simulink model "gm_uz_pmsm_model_9ph_vnl"  (R2021b)
settings: Solver=FixedStepAuto  StartTime=0.0  StopTime=0.8  RelTol=1e-3
PreLoadFcn:
  | uz_pmsm_model_9ph_init_parameter
undefined symbols (not defined in the file or in its folder): a, b, c, friction_coefficient, inertia, k_i_d, k_i_q, k_p_d, k_p_q, Kpd, L_d, L_o1, L_o2, L_q, L_x1, L_x2, L_y1, L_y2, L_zero, polepair, psi_pm, R_1, static_friction_torque, Tnd, ts
libraries: hdlmdlgenlib x191, hdlsllib x90, dspsigops x19, simulink x17, slpidlib x2, spsAlphaBetaZerotodq0Lib x1, pid_lib x1, spsdq0toAlphaBetaZeroLib x1
(part 2 of 7)

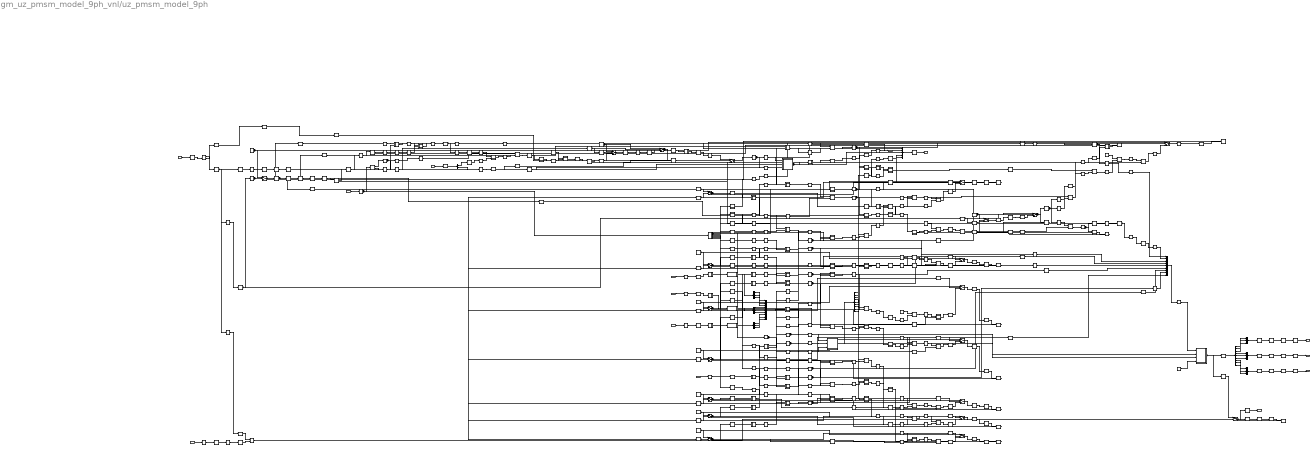
== system gm_uz_pmsm_model_9ph_vnl/uz_pmsm_model_9ph ==
  note: PMSM electric and magentic
  note: Mechanical
  note: Outputs
  note: Inputs
  note: o1 equation
  note: DQ equations
  note: o2 equation
  note: x1 equation
  note: y1 equation
  note: x2 equation
  note: y2 equation
  note: zero equation
  note: load torque negative!!!
  Model_Parameter : Inport  SampleTime=2e-06
  physical_parameters : Inport  Port=2  SampleTime=2e-06
  input : Inport  Port=3  OutDataTypeStr=single  PortDimensions=[2]  SampleTime=2e-06
  u_abc1_pl : Inport  Port=4  OutDataTypeStr=fixdt(1, 25, 12)  PortDimensions=[3]  SampleTime=2e-06
  u_abc2_pl : Inport  Port=5  OutDataTypeStr=fixdt(1, 25, 12)  PortDimensions=[3]  SampleTime=2e-06
  u_abc3_pl : Inport  Port=6  OutDataTypeStr=fixdt(1, 25, 12)  PortDimensions=[3]  SampleTime=2e-06
  in_theta_el : Inport  Port=7  OutDataTypeStr=fixdt(1, 25, 12)  PortDimensions=1  SampleTime=2e-06
  pwm_trig : Inport  Port=8  OutDataTypeStr=boolean  PortDimensions=1  SampleTime=2e-06
  Add : Subsystem
      mask Display: disp('NFP\nadd');
  Add1 : Subsystem
      mask Display: disp('NFP\nadd');
  Add1_outbuff : hdlmdlgenlib/Buffer
      settings: SourceProductBaseCode=SL
  Add2 : Subsystem
      mask Display: disp('NFP\nadd');
  Add2_outbuff : hdlmdlgenlib/Buffer
      settings: SourceProductBaseCode=SL
  Add3 : Subsystem
      mask Display: disp('NFP\nadd');
  Add3_outbuff : hdlmdlgenlib/Buffer
      settings: SourceProductBaseCode=SL
  Add4 : Subsystem
      mask Display: disp('NFP\nadd');
  Add4_outbuff : hdlmdlgenlib/Buffer
      settings: SourceProductBaseCode=SL
  Add5 : Subsystem
      mask Display: disp('NFP\nadd');
  Add5_outbuff : hdlmdlgenlib/Buffer
      settings: SourceProductBaseCode=SL
  Add6 : Subsystem
      mask Display: disp('NFP\nadd');
  Add6_outbuff : hdlmdlgenlib/Buffer
      settings: SourceProductBaseCode=SL
  Add_outbuff : hdlmdlgenlib/Buffer
      settings: SourceProductBaseCode=SL
  Cast To Double : Subsystem
      mask Display: disp('NFP\nconv');
  Cast To Double1 : Subsystem
      mask Display: disp('NFP\nconv');
  Cast To Double2 : Subsystem
      mask Display: disp('NFP\nconv');
  Data Type Conversion1 : Subsystem
      mask Display: disp('NFP\nconv');
  Data Type Conversion11 : Subsystem
      mask Display: disp('NFP\nconv');
  Data Type Conversion12 : Subsystem
      mask Display: disp('NFP\nconv');
  Data Type Conversion13 : Subsystem
      mask Display: disp('NFP\nconv');
  Data Type Conversion13_outbuff : hdlmdlgenlib/Buffer
      settings: SourceProductBaseCode=SL
  Data Type Conversion14 : Subsystem
      mask Display: disp('NFP\nconv');
  Data Type Conversion141 : Subsystem
      mask Display: disp('NFP\nconv');
  Data Type Conversion14_outbuff : hdlmdlgenlib/Buffer
      settings: SourceProductBaseCode=SL
  Data Type Conversion15 : Subsystem
      mask Display: disp('NFP\nconv');
  Data Type Conversion15_outbuff : hdlmdlgenlib/Buffer
      settings: SourceProductBaseCode=SL
  Data Type Conversion16 : Subsystem
      mask Display: disp('NFP\nconv');
  Data Type Conversion16_outbuff : hdlmdlgenlib/Buffer
      settings: SourceProductBaseCode=SL
  Data Type Conversion17 : Subsystem
      mask Display: disp('NFP\nconv');
  Data Type Conversion17_outbuff : hdlmdlgenlib/Buffer
      settings: SourceProductBaseCode=SL
  Data Type Conversion18 : Subsystem
      mask Display: disp('NFP\nconv');
  Data Type Conversion18_outbuff : hdlmdlgenlib/Buffer
      settings: SourceProductBaseCode=SL
  Data Type Conversion19 : Subsystem
      mask Display: disp('NFP\nconv');
  Data Type Conversion19_outbuff : hdlmdlgenlib/Buffer
      settings: SourceProductBaseCode=SL
  Data Type Conversion1_outbuff : hdlmdlgenlib/Buffer
      settings: SourceProductBaseCode=SL
  Data Type Conversion20 : Subsystem
      mask Display: disp('NFP\nconv');
  Data Type Conversion20_outbuff : hdlmdlgenlib/Buffer
      settings: SourceProductBaseCode=SL
  Data Type Conversion21 : Subsystem
      mask Display: disp('NFP\nconv');
  Data Type Conversion22 : Subsystem
      mask Display: disp('NFP\nconv');
  Data Type Conversion23 : Subsystem
      mask Display: disp('NFP\nconv');
  Data Type Conversion23_outbuff : hdlmdlgenlib/Buffer
      settings: SourceProductBaseCode=SL
  Data Type Conversion24 : Subsystem
      mask Display: disp('NFP\nconv');
  Data Type Conversion24_outbuff : hdlmdlgenlib/Buffer
      settings: SourceProductBaseCode=SL
  Data Type Conversion25 : Subsystem
      mask Display: disp('NFP\nconv');
  Data Type Conversion25_outbuff : hdlmdlgenlib/Buffer
      settings: SourceProductBaseCode=SL
  Data Type Conversion26 : Subsystem
      mask Display: disp('NFP\nconv');
  Data Type Conversion26_outbuff : hdlmdlgenlib/Buffer
      settings: SourceProductBaseCode=SL
  Data Type Conversion27 : Subsystem
      mask Display: disp('NFP\nconv');
  Data Type Conversion27_outbuff : hdlmdlgenlib/Buffer
      settings: SourceProductBaseCode=SL
  Data Type Conversion28 : Subsystem
      mask Display: disp('NFP\nconv');
  Data Type Conversion28_outbuff : hdlmdlgenlib/Buffer
      settings: SourceProductBaseCode=SL
  Data Type Conversion29 : Subsystem
      mask Display: disp('NFP\nconv');
  Data Type Conversion29_outbuff : hdlmdlgenlib/Buffer
      settings: SourceProductBaseCode=SL
  Data Type Conversion3 : Subsystem
      mask Display: disp('NFP\nconv');
  Data Type Conversion30 : Subsystem
      mask Display: disp('NFP\nconv');
  Data Type Conversion30_outbuff : hdlmdlgenlib/Buffer
      settings: SourceProductBaseCode=SL
  Data Type Conversion31 : Subsystem
      mask Display: disp('NFP\nconv');
  Data Type Conversion31_outbuff : hdlmdlgenlib/Buffer
      settings: SourceProductBaseCode=SL
  Data Type Conversion32 : Subsystem
      mask Display: disp('NFP\nconv');
  Data Type Conversion32_outbuff : hdlmdlgenlib/Buffer
      settings: SourceProductBaseCode=SL
  Data Type Conversion33 : Subsystem
      mask Display: disp('NFP\nconv');
  Data Type Conversion331 : Subsystem
      mask Display: disp('NFP\nconv');
  Data Type Conversion33_outbuff : hdlmdlgenlib/Buffer
      settings: SourceProductBaseCode=SL
  Data Type Conversion33_outbuff1 : hdlmdlgenlib/Buffer
      settings: SourceProductBaseCode=SL
  Data Type Conversion34 : DataTypeConversion  OutDataTypeStr=fixdt(1, 25, 12)  RndMeth=Nearest  SampleTime=1e-08
  Data Type Conversion37 : Subsystem
      mask Display: disp('NFP\nconv');
  Data Type Conversion5 : Subsystem
      mask Display: disp('NFP\nconv');
  Data Type Conversion51 : Subsystem
      mask Display: disp('NFP\nconv');
  Data Type Conversion8 : DataTypeConversion  OutDataTypeStr=boolean  RndMeth=Nearest  SampleTime=2e-06
  Data Type Conversion81 : Subsystem
      mask Display: disp('NFP\nconv');
  Data Type Conversion8_outbuff : hdlmdlgenlib/Buffer
      settings: SourceProductBaseCode=SL
  Data Type Conversion9 : Subsystem
      mask Display: disp('NFP\nconv');
  Delay{,1..3} (4 alike) : Delay  DelayLength=double(2)  InitialCondition=0  SampleTime=2e-06
  Delay1_lowered{,1..9} (10 alike) : RateTransition  OutPortSampleTimeOpt=Multiple of input port sample time  OutPortSampleTimeMultiple=200
  Delay4 : Delay  DelayLength=double(1)  InitialCondition=0  SampleTime=2e-06
  Delay{7..9,41,51,61} (6 alike) : RateTransition  OutPortSampleTimeOpt=Multiple of input port sample time  OutPortSampleTimeMultiple=200
  Delay5 : Delay  DelayLength=double(1)  InitialCondition=0  SampleTime=2e-06
  Delay6 : Delay  DelayLength=double(1)  InitialCondition=0  SampleTime=2e-06
  Demux1_mux_1 : Mux  Inputs=3
  Demux1_mux_2 : Mux  Inputs=3
  Demux1_mux_3 : Mux  Inputs=3
  Divide : Subsystem
      mask Display: disp('NFP\nmul');
  Divide1 : Subsystem
      mask Display: disp('NFP\nmul');
  Divide10 : Subsystem
      mask Display: disp('NFP\nmul');
  Divide10_outbuff : hdlmdlgenlib/Buffer
      settings: SourceProductBaseCode=SL
  Divide11 : Subsystem
      mask Display: disp('NFP\nmul');
  Divide11_outbuff : hdlmdlgenlib/Buffer
      settings: SourceProductBaseCode=SL
  Divide12 : Subsystem
      mask Display: disp('NFP\nmul');
  Divide12_outbuff : hdlmdlgenlib/Buffer
      settings: SourceProductBaseCode=SL
  Divide13 : Subsystem
      mask Display: disp('NFP\nmul');
  Divide13_outbuff : hdlmdlgenlib/Buffer
      settings: SourceProductBaseCode=SL
  Divide1_outbuff : hdlmdlgenlib/Buffer
      settings: SourceProductBaseCode=SL
  Divide2 : Subsystem
      mask Display: disp('NFP\nmul');
  Divide2_outbuff : hdlmdlgenlib/Buffer
      settings: SourceProductBaseCode=SL
  Divide3 : Subsystem
      mask Display: disp('NFP\nmul');
  Divide3_outbuff : hdlmdlgenlib/Buffer
      settings: SourceProductBaseCode=SL
  Divide4 : Subsystem
      mask Display: disp('NFP\nmul');
  Divide4_outbuff : hdlmdlgenlib/Buffer
      settings: SourceProductBaseCode=SL
  Divide5 : Subsystem
      mask Display: disp('NFP\nmul');
  Divide5_outbuff : hdlmdlgenlib/Buffer
      settings: SourceProductBaseCode=SL
  Divide6 : Subsystem
      mask Display: disp('NFP\nmul');
  Divide6_outbuff : hdlmdlgenlib/Buffer
      settings: SourceProductBaseCode=SL
  Divide7 : Subsystem
      mask Display: disp('NFP\nmul');
  Divide7_outbuff : hdlmdlgenlib/Buffer
      settings: SourceProductBaseCode=SL
  Divide8 : Subsystem
      mask Display: disp('NFP\nmul');
  Divide8_outbuff : hdlmdlgenlib/Buffer
      settings: SourceProductBaseCode=SL
  Divide9 : Subsystem
      mask Display: disp('NFP\nmul');
  Divide9_outbuff : hdlmdlgenlib/Buffer
      settings: SourceProductBaseCode=SL
  Divide_outbuff : hdlmdlgenlib/Buffer
      settings: SourceProductBaseCode=SL
  Factor : Subsystem
      mask Display: disp('NFP\nmul');
  Factor_const : Constant  Value=single(4.5)  OutDataTypeStr=single  SampleTime=1e-08
  Factor_outbuff : hdlmdlgenlib/Buffer
      settings: SourceProductBaseCode=SL
  From{,1..24,26..27,30..31,41,51,61,71,81,91,101,111,121,131,141,151,181,191,211,311} (45 alike) : hdlmdlgenlib/Buffer
      settings: SourceProductBaseCode=SL
  Gain : Subsystem
      mask Display: disp('NFP\nmul');
  Gain1 : Subsystem
      mask Display: disp('NFP\nmul');
  Gain2 : Subsystem
      mask Display: disp('NFP\nmul');
  Gain3 : Subsystem
      mask Display: disp('NFP\nmul');
  Gain4 : Subsystem
      mask Display: disp('NFP\nmul');
  Gain5 : Subsystem
      mask Display: disp('NFP\nmul');
  Gain6 : Subsystem
      mask Display: disp('NFP\nmul');
  Gain7 : Subsystem
      mask Display: disp('NFP\nmul');
  Gain8 : Subsystem
      mask Display: disp('NFP\nmul');
  Gain9 : Subsystem
      mask Display: disp('NFP\nmul');
  Gain_const{,1..9} (10 alike) : Constant  Value=double(2e-06)  OutDataTypeStr=double  SampleTime=1e-08
  Gain_outbuff{,1..9} (10 alike) : hdlmdlgenlib/Buffer
      settings: SourceProductBaseCode=SL
  Goto{,1..7,9..16,32..36,91,111,121,131,141,151} (27 alike) : hdlmdlgenlib/Buffer
      settings: SourceProductBaseCode=SL
  Initial_Val{,1..9} (10 alike) : Constant  Value=double(0)  OutDataTypeStr=double  SampleTime=1e-08
  Line-Line to Phase voltage : Subsystem
  Line-Line to Phase voltage1 : Subsystem
  Line-Line to Phase voltage2 : Subsystem
  Logical Operator : Logic  Operator=OR  AllPortsSameDT=off  OutDataTypeStr=boolean  SampleTime=1e-08
  M_Mi : hdlmdlgenlib/Buffer
      settings: SourceProductBaseCode=SL
  Product : Subsystem
      mask Display: disp('NFP\nmul');
  Product1 : Subsystem
      mask Display: disp('NFP\nmul');
  Product10 : Subsystem
      mask Display: disp('NFP\nmul');
  Product10_outbuff : hdlmdlgenlib/Buffer
      settings: SourceProductBaseCode=SL
  Product11 : Subsystem
      mask Display: disp('NFP\nmul');
  Product11_outbuff : hdlmdlgenlib/Buffer
      settings: SourceProductBaseCode=SL
  Product1_outbuff : hdlmdlgenlib/Buffer
      settings: SourceProductBaseCode=SL
  Product2 : Subsystem
      mask Display: disp('NFP\nmul');
  Product2_outbuff : hdlmdlgenlib/Buffer
      settings: SourceProductBaseCode=SL
  Product3 : Subsystem
      mask Display: disp('NFP\nmul');
  Product3_outbuff : hdlmdlgenlib/Buffer
      settings: SourceProductBaseCode=SL
  Product5 : Subsystem
      mask Display: disp('NFP\nmul');
  Product5_outbuff : hdlmdlgenlib/Buffer
      settings: SourceProductBaseCode=SL
  Product6 : Subsystem
      mask Display: disp('NFP\nmul');
  Product6_outbuff : hdlmdlgenlib/Buffer
      settings: SourceProductBaseCode=SL
  Product7 : Subsystem
      mask Display: disp('NFP\nmul');
  Product7_outbuff : hdlmdlgenlib/Buffer
      settings: SourceProductBaseCode=SL
  Product8 : Subsystem
      mask Display: disp('NFP\nmul');
  Product8_outbuff : hdlmdlgenlib/Buffer
      settings: SourceProductBaseCode=SL
  Product9 : Subsystem
      mask Display: disp('NFP\nmul');
  Product9_outbuff : hdlmdlgenlib/Buffer
      settings: SourceProductBaseCode=SL
  Product_outbuff : hdlmdlgenlib/Buffer
      settings: SourceProductBaseCode=SL
  Sine_Cosine : Subsystem
      mask Display: disp('NFP\ntrig2');
  Sum1 : Subsystem
      mask Display: disp('NFP\nadd');
  Sum1_outbuff : hdlmdlgenlib/Buffer
      settings: SourceProductBaseCode=SL
  Sum1_stage2 : Subsystem
      mask Display: disp('NFP\nadd');
  Sum1_stage2_outbuff : hdlmdlgenlib/Buffer
      settings: SourceProductBaseCode=SL
  Sum1_stage3 : Subsystem
      mask Display: disp('NFP\nadd');
  Sum1_stage3_outbuff : hdlmdlgenlib/Buffer
      settings: SourceProductBaseCode=SL
  Sum2 : Subsystem
      mask Display: disp('NFP\nadd');
  Sum2_outbuff : hdlmdlgenlib/Buffer
      settings: SourceProductBaseCode=SL
  Sum3 : Subsystem
      mask Display: disp('NFP\nadd');
  Sum31 : Subsystem
      mask Display: disp('NFP\nadd');
  Sum310 : Subsystem
      mask Display: disp('NFP\nadd');
  Sum32 : Subsystem
      mask Display: disp('NFP\nadd');
  Sum33 : Subsystem
      mask Display: disp('NFP\nadd');
  Sum34 : Subsystem
      mask Display: disp('NFP\nadd');
  Sum35 : Subsystem
      mask Display: disp('NFP\nadd');
  Sum36 : Subsystem
      mask Display: disp('NFP\nadd');
  Sum37 : Subsystem
      mask Display: disp('NFP\nadd');
  Sum38 : Subsystem
      mask Display: disp('NFP\nadd');
  Sum39 : Subsystem
      mask Display: disp('NFP\nadd');
  Sum3_outbuff{,1..10} (11 alike) : hdlmdlgenlib/Buffer
      settings: SourceProductBaseCode=SL
  Sum_stage2 : Subsystem
      mask Display: disp('NFP\nadd');
  Sum_stage2_outbuff : hdlmdlgenlib/Buffer
      settings: SourceProductBaseCode=SL
  Sum_stage3 : Subsystem
      mask Display: disp('NFP\nadd');
  Sum_stage3_outbuff : hdlmdlgenlib/Buffer
      settings: SourceProductBaseCode=SL
  Switch : Switch  Criteria=u2 ~= 0  Threshold=double(0)  OutDataTypeStr=single  SampleTime=1e-08
  Switch1 : Switch  Criteria=u2 ~= 0  Threshold=double(0)  OutDataTypeStr=single  SampleTime=1e-08
  Transformation : Subsystem
  Transformation1 : Subsystem
  Transformation_out1_0_wire : hdlmdlgenlib/Buffer
      settings: SourceProductBaseCode=SL
  Transformation_out1_1_wire : hdlmdlgenlib/Buffer
      settings: SourceProductBaseCode=SL
  Wrapped State DTI : Subsystem
  bus_selector : BusSelector  OutputSignals=1_L_d,1_L_q,R_1,polepair,psi_pm,L_z1,L_z2,L_x1,L_y1,L_x2,L_y2,L_z3
  bus_selector1 : BusSelector  OutputSignals=reset_integrators,simulate_mechanical
  bus_selector2 : BusSelector  OutputSignals=polepair,1_J
  crp_out_delay{,1..15} (16 alike) : Delay  DelayLength=double(1)  InitialCondition=0  SampleTime=1e-08
  ctr_199 : simulink/Sources/Counter Limited  uplimit=double(199)  tsamp=1e-08
  delay : Delay  DelayLength=double(1)  InitialCondition=0  SampleTime=2e-06
  delayMatch{,67..70} (5 alike) : Delay  DelayLength=double(1)  InitialCondition=0  SampleTime=2e-06
  delayMatch{1..19,21,29..32,35,41,43,45,47,49,51,53,64..66} (35 alike) : Delay  DelayLength=double(1)  InitialCondition=0  SampleTime=1e-08
  delayMatch20 : Delay  DelayLength=double(27)  InitialCondition=0  SampleTime=1e-08
  delayMatch22 : Delay  DelayLength=double(54)  InitialCondition=0  SampleTime=1e-08
  delayMatch23 : Delay  DelayLength=double(54)  InitialCondition=0  SampleTime=1e-08
  delayMatch24 : Delay  DelayLength=double(72)  InitialCondition=0  SampleTime=1e-08
  delayMatch25 : Delay  DelayLength=double(21)  InitialCondition=0  SampleTime=1e-08
  delayMatch{26..28,33,40,42,44,46,48,50,52} (11 alike) : Delay  DelayLength=double(3)  InitialCondition=0  SampleTime=1e-08
  delayMatch34 : Delay  DelayLength=double(6)  InitialCondition=0  SampleTime=1e-08
  delayMatch{36,55..61} (8 alike) : Delay  DelayLength=double(9)  InitialCondition=0  SampleTime=1e-08
  delayMatch37 : Delay  DelayLength=double(15)  InitialCondition=0  SampleTime=1e-08
  delayMatch38 : Delay  DelayLength=double(6)  InitialCondition=0  SampleTime=1e-08
  delayMatch39 : Delay  DelayLength=double(36)  InitialCondition=0  SampleTime=1e-08
  delayMatch54 : Delay  DelayLength=double(6)  InitialCondition=0  SampleTime=1e-08
  delayMatch62 : Delay  DelayLength=double(15)  InitialCondition=0  SampleTime=1e-08
  delayMatch63 : Delay  DelayLength=double(60)  InitialCondition=0  SampleTime=1e-08
  i_d : hdlmdlgenlib/Buffer
      settings: SourceProductBaseCode=SL
  i_q : hdlmdlgenlib/Buffer
      settings: SourceProductBaseCode=SL
  in0_repeat : RateTransition  Integrity=off  Deterministic=off  OutPortSampleTimeOpt=Multiple of input port sample time  OutPortSampleTimeMultiple=1/200
  in10_repeat : dspsigops/Repeat  N=double(200)  RateOptions=Allow multirate processing  ic=0  mode=Unused parameter value
  in11_repeat : dspsigops/Repeat  N=double(200)  RateOptions=Allow multirate processing  ic=0  mode=Unused parameter value
  in12_repeat : dspsigops/Repeat  N=double(200)  RateOptions=Allow multirate processing  ic=0  mode=Unused parameter value
  in13_repeat : dspsigops/Repeat  N=double(200)  RateOptions=Allow multirate processing  ic=0  mode=Unused parameter value
  in14_repeat : dspsigops/Repeat  N=double(200)  RateOptions=Allow multirate processing  ic=0  mode=Unused parameter value
  in15_repeat : dspsigops/Repeat  N=double(200)  RateOptions=Allow multirate processing  ic=0  mode=Unused parameter value
  in16_repeat : dspsigops/Repeat  N=double(200)  RateOptions=Allow multirate processing  ic=0  mode=Unused parameter value
  in17_repeat : dspsigops/Repeat  N=double(200)  RateOptions=Allow multirate processing  ic=0  mode=Unused parameter value
  in1_repeat : RateTransition  Integrity=off  Deterministic=off  OutPortSampleTimeOpt=Multiple of input port sample time  OutPortSampleTimeMultiple=1/200
  in1_repeat1 : dspsigops/Repeat  N=double(200)  RateOptions=Allow multirate processing  ic=0  mode=Unused parameter value
  in2_repeat : dspsigops/Repeat  N=double(200)  RateOptions=Allow multirate processing  ic=0  mode=Unused parameter value
  in3_repeat : dspsigops/Repeat  N=double(200)  RateOptions=Allow multirate processing  ic=0  mode=Unused parameter value
  in3_repeat1 : dspsigops/Repeat  N=double(200)  RateOptions=Allow multirate processing  ic=0  mode=Unused parameter value
  in4_repeat : dspsigops/Repeat  N=double(200)  RateOptions=Allow multirate processing  ic=0  mode=Unused parameter value
  in5_repeat : dspsigops/Repeat  N=double(200)  RateOptions=Allow multirate processing  ic=0  mode=Unused parameter value
  in6_repeat : dspsigops/Repeat  N=double(200)  RateOptions=Allow multirate processing  ic=0  mode=Unused parameter value
  in7_repeat : dspsigops/Repeat  N=double(200)  RateOptions=Allow multirate processing  ic=0  mode=Unused parameter value
  in8_repeat : dspsigops/Repeat  N=double(200)  RateOptions=Allow multirate processing  ic=0  mode=Unused parameter value
  in9_repeat : dspsigops/Repeat  N=double(200)  RateOptions=Allow multirate processing  ic=0  mode=Unused parameter value
  integrator_out1 : hdlmdlgenlib/Buffer
      settings: SourceProductBaseCode=SL
  mechanical_system_out1 : hdlmdlgenlib/Buffer
      settings: SourceProductBaseCode=SL
  mux : Mux  Inputs=5
  mux1 : Mux  Inputs=9
  mux2 : Mux  Inputs=9
  pmsm_out3 : hdlmdlgenlib/Buffer
      settings: SourceProductBaseCode=SL
  pmsm_out4 : hdlmdlgenlib/Buffer
      settings: SourceProductBaseCode=SL
  psi_{,1..6} (7 alike) : hdlmdlgenlib/Buffer
      settings: SourceProductBaseCode=SL
  psi_d : hdlmdlgenlib/Buffer
      settings: SourceProductBaseCode=SL
  psi_q : hdlmdlgenlib/Buffer
      settings: SourceProductBaseCode=SL
  reset_in{,1..9} (10 alike) : Switch  Criteria=u2 ~= 0  Threshold=double(0)  OutDataTypeStr=double  SampleTime=1e-08
  reset_out{,1..9} (10 alike) : Switch  Criteria=u2 ~= 0  Threshold=double(0)  OutDataTypeStr=double  SampleTime=1e-08
  t : RateTransition  OutPortSampleTimeOpt=Multiple of input port sample time  OutPortSampleTimeMultiple=200
  t1 : Demux  Outputs=3
  t2 : Demux  Outputs=3
  t3 : Demux  Outputs=3
  t4 : Demux  Outputs=9
  t5 : Demux  Outputs=2
  t6 : Demux  Outputs=9
  t7 : RateTransition  OutPortSampleTimeOpt=Multiple of input port sample time  OutPortSampleTimeMultiple=200
  outputs : Outport  SampleTime=2e-06
  i_abc_ps : Outport  Port=2  SampleTime=2e-06
  i_abc1_pl : Outport  Port=3  SampleTime=2e-06
  i_abc2_pl : Outport  Port=4  SampleTime=2e-06
  i_abc3_pl : Outport  Port=5  SampleTime=2e-06
  out_theta_el : Outport  Port=6  SampleTime=2e-06
  wires:
  delayMatch66/1 -> Switch/3
  delayMatch65/1 -> Logical Operator/2
  Logical Operator/1 -> Switch/2
  in3_repeat1/1 -> delayMatch66/1
  in1_repeat1/1 -> delayMatch65/1
  crp_out_delay15/1 -> Delay9/1
  Switch/1 -> crp_out_delay15/1, t7/1
  ctr_199/1 -> Transformation1/4(enb_counter)
  delayMatch63/1 -> delayMatch64/1
  reset_in9/1 -> crp_out_delay11/1
  reset_in8/1 -> crp_out_delay10/1
  reset_in7/1 -> crp_out_delay9/1
  reset_in6/1 -> crp_out_delay8/1
  reset_in5/1 -> crp_out_delay7/1
  reset_in4/1 -> crp_out_delay6/1
  reset_in3/1 -> crp_out_delay5/1
  delayMatch24/1 -> delayMatch63/1
  mux2/1 -> delayMatch62/1
  From81/1 -> delayMatch54/1
  From30/1 -> delayMatch53/1
  From211/1 -> delayMatch52/1
  From26/1 -> delayMatch51/1
  From20/1 -> delayMatch50/1
  From22/1 -> delayMatch49/1
  From17/1 -> delayMatch48/1
  From181/1 -> delayMatch47/1
  From16/1 -> delayMatch46/1
  From141/1 -> delayMatch45/1
  From13/1 -> delayMatch44/1
  From8/1 -> delayMatch43/1
  From121/1 -> delayMatch42/1
  From41/1 -> delayMatch41/1
  From111/1 -> delayMatch40/1
  From/1 -> delayMatch39/1
  Product3_outbuff/1 -> delayMatch38/1
  pmsm_out4/1 -> delayMatch37/1
  pmsm_out3/1 -> delayMatch36/1
  psi_q/1 -> Data Type Conversion13/1(In1), delayMatch28/1, delayMatch35/1
  Data Type Conversion33_outbuff/1 -> Product8/2(In2), Product7/2(In2)
  From10/1 -> delayMatch34/1
  psi_d/1 -> Data Type Conversion23/1(In1), delayMatch29/1, delayMatch33/1
  From4/1 -> reset_out1/2, delayMatch32/1
  reset_out1/1 -> integrator_out1/1, delayMatch31/1
  From15/1 -> delayMatch30/1
  delayMatch33/1 -> Sum2/1(In1)
  delayMatch35/1 -> Product/2(In2)
  From6/1 -> Product10/2(In2)
  From21/1 -> delayMatch27/1
  From14/1 -> delayMatch26/1
  Gain9/1(Out1) -> Gain_outbuff9/1
  Gain8/1(Out1) -> Gain_outbuff8/1
  Gain7/1(Out1) -> Gain_outbuff7/1
  Gain6/1(Out1) -> Gain_outbuff6/1
  Gain5/1(Out1) -> Gain_outbuff5/1
  Gain4/1(Out1) -> Gain_outbuff4/1
  Gain3/1(Out1) -> Gain_outbuff3/1
  Factor/1(Out1) -> Factor_outbuff/1
  Gain2/1(Out1) -> Gain_outbuff2/1
  Gain1/1(Out1) -> Gain_outbuff1/1
  Gain/1(Out1) -> Gain_outbuff/1
  Data Type Conversion51/1(Out1) -> Switch/1
  Divide13/1(Out1) -> Divide13_outbuff/1
  Data Type Conversion20/1(Out1) -> Data Type Conversion20_outbuff/1
  Sum310/1(Out1) -> Sum3_outbuff10/1
  Data Type Conversion30/1(Out1) -> Data Type Conversion30_outbuff/1
  Add6/1(Out1) -> Add6_outbuff/1
  Divide12/1(Out1) -> Divide12_outbuff/1
  Divide11/1(Out1) -> Divide11_outbuff/1
  Data Type Conversion19/1(Out1) -> Data Type Conversion19_outbuff/1
  Sum39/1(Out1) -> Sum3_outbuff9/1
  Data Type Conversion29/1(Out1) -> Data Type Conversion29_outbuff/1
  Add5/1(Out1) -> Add5_outbuff/1
  Divide10/1(Out1) -> Divide10_outbuff/1
  Divide9/1(Out1) -> Divide9_outbuff/1
  Data Type Conversion18/1(Out1) -> Data Type Conversion18_outbuff/1
  Sum38/1(Out1) -> Sum3_outbuff8/1
  Data Type Conversion28/1(Out1) -> Data Type Conversion28_outbuff/1
  Add4/1(Out1) -> Add4_outbuff/1
  Divide8/1(Out1) -> Divide8_outbuff/1
  Divide7/1(Out1) -> Divide7_outbuff/1
  Data Type Conversion17/1(Out1) -> Data Type Conversion17_outbuff/1
  Sum37/1(Out1) -> Sum3_outbuff7/1
  Data Type Conversion27/1(Out1) -> Data Type Conversion27_outbuff/1
  Add3/1(Out1) -> Add3_outbuff/1
  Divide6/1(Out1) -> Divide6_outbuff/1
  Divide5/1(Out1) -> Divide5_outbuff/1
  Data Type Conversion16/1(Out1) -> Data Type Conversion16_outbuff/1
  Sum36/1(Out1) -> Sum3_outbuff6/1
  Data Type Conversion26/1(Out1) -> Data Type Conversion26_outbuff/1
  Add2/1(Out1) -> Add2_outbuff/1
  Divide4/1(Out1) -> Divide4_outbuff/1
  Divide3/1(Out1) -> Divide3_outbuff/1
  Data Type Conversion15/1(Out1) -> Data Type Conversion15_outbuff/1
  Sum35/1(Out1) -> Sum3_outbuff5/1
  Data Type Conversion25/1(Out1) -> Data Type Conversion25_outbuff/1
  Add1/1(Out1) -> Add1_outbuff/1
  Divide2/1(Out1) -> Divide2_outbuff/1
  Divide1/1(Out1) -> Divide1_outbuff/1
  Data Type Conversion141/1(Out1) -> Data Type Conversion14_outbuff/1
  Sum34/1(Out1) -> Sum3_outbuff4/1
  Data Type Conversion24/1(Out1) -> Data Type Conversion24_outbuff/1
  Add/1(Out1) -> Add_outbuff/1
  Divide/1(Out1) -> Divide_outbuff/1
  Product9/1(Out1) -> Product9_outbuff/1
  Sum33/1(Out1) -> Sum3_outbuff3/1
  Product2/1(Out1) -> Product2_outbuff/1
  Data Type Conversion32/1(Out1) -> Data Type Conversion32_outbuff/1
  Product5/1(Out1) -> Product5_outbuff/1
  Sum2/1(Out1) -> Sum2_outbuff/1
  Sum32/1(Out1) -> Sum3_outbuff2/1
  Sum_stage3/1(Out1) -> Sum_stage3_outbuff/1
  Sum_stage2/1(Out1) -> Sum_stage2_outbuff/1
  Product8/1(Out1) -> Product8_outbuff/1
  Product/1(Out1) -> Product_outbuff/1
  Product10/1(Out1) -> Product10_outbuff/1
  Data Type Conversion331/1(Out1) -> Data Type Conversion33_outbuff1/1
  Data Type Conversion81/1(Out1) -> Data Type Conversion8_outbuff/1
  Sum31/1(Out1) -> Sum3_outbuff1/1
  Data Type Conversion14/1(Out1) -> Data Type Conversion1_outbuff/1
  Product11/1(Out1) -> Product11_outbuff/1
  Sum1/1(Out1) -> Sum1_outbuff/1
  Sum3/1(Out1) -> Sum3_outbuff/1
  Sum1_stage3/1(Out1) -> Sum1_stage3_outbuff/1
  Sum1_stage2/1(Out1) -> Sum1_stage2_outbuff/1
  Product1/1(Out1) -> Product1_outbuff/1
  Product7/1(Out1) -> Product7_outbuff/1
  Product6/1(Out1) -> Product6_outbuff/1
  Data Type Conversion13/1(Out1) -> Data Type Conversion13_outbuff/1
  Product3/1(Out1) -> Product3_outbuff/1
  Data Type Conversion23/1(Out1) -> Data Type Conversion23_outbuff/1
  Data Type Conversion31/1(Out1) -> Data Type Conversion31_outbuff/1
  Data Type Conversion12/1(Out1) -> Goto35/1
  Data Type Conversion22/1(Out1) -> Sum1_stage2/1(In1)
  Data Type Conversion3/1(Out1) -> Goto34/1
  Data Type Conversion21/1(Out1) -> Sum_stage2/1(In1)
  Sine_Cosine/2(Out2) -> Goto16/1
  Sine_Cosine/1(Out1) -> Goto15/1
  Data Type Conversion37/1(Out1) -> Sine_Cosine/1(In1)
  Data Type Conversion9/1(Out1) -> delayMatch25/1
  Cast To Double2/1(Out1) -> Line-Line to Phase voltage2/1(In1)
  Cast To Double1/1(Out1) -> Line-Line to Phase voltage1/1(In1)
  Cast To Double/1(Out1) -> Line-Line to Phase voltage/1(In1)
  Data Type Conversion33/1(Out1) -> Data Type Conversion33_outbuff/1
  Data Type Conversion5/1(Out1) -> Goto33/1
  Data Type Conversion11/1(Out1) -> Goto36/1
  delayMatch20/1 -> delayMatch24/1
  delayMatch18/1 -> reset_in9/2
  delayMatch17/1 -> Sum310/2(In2)
  delayMatch16/1 -> reset_in8/2
  delayMatch15/1 -> Sum39/2(In2)
  delayMatch14/1 -> reset_in7/2
  delayMatch13/1 -> Sum38/2(In2)
  delayMatch12/1 -> reset_in6/2
  delayMatch11/1 -> Sum37/2(In2)
  delayMatch10/1 -> reset_in5/2
  delayMatch9/1 -> Sum36/2(In2)
  delayMatch8/1 -> reset_in4/2
  delayMatch7/1 -> Sum35/2(In2)
  delayMatch6/1 -> reset_in3/2
  delayMatch5/1 -> Sum34/2(In2)
  delayMatch4/1 -> reset_in2/2
  delayMatch3/1 -> Sum32/2(In2)
  delayMatch2/1 -> reset_in/2
  delayMatch1/1 -> Sum3/2(In2)
  Goto16/1 -> Transformation1/3(cos_theta_el), delayMatch23/1
  Goto15/1 -> Transformation1/2(sin_theta_el), delayMatch22/1
  Demux1_mux_3/1 -> crp_out_delay14/1
  Demux1_mux_2/1 -> crp_out_delay13/1
  Demux1_mux_1/1 -> crp_out_delay12/1
  From131/1 -> delayMatch21/1
  From11/1 -> delayMatch20/1
  From5/1 -> delayMatch19/1
  M_Mi/1 -> crp_out_delay4/1, Goto7/1
  reset_in1/1 -> crp_out_delay2/1
  From311/1 -> reset_out9/2, delayMatch18/1
  reset_out9/1 -> psi_6/1, delayMatch17/1
  Divide12_outbuff/1 -> Add6/2(In2)
  From27/1 -> reset_out8/2, delayMatch16/1
  reset_out8/1 -> psi_5/1, delayMatch15/1
  Divide10_outbuff/1 -> Add5/2(In2)
  From23/1 -> reset_out7/2, delayMatch14/1
  reset_out7/1 -> psi_4/1, delayMatch13/1
  Divide8_outbuff/1 -> Add4/2(In2)
  From191/1 -> reset_out6/2, delayMatch12/1
  reset_out6/1 -> psi_3/1, delayMatch11/1
  Divide6_outbuff/1 -> Add3/2(In2)
  From151/1 -> reset_out5/2, delayMatch10/1
  reset_out5/1 -> psi_2/1, delayMatch9/1
  Divide4_outbuff/1 -> Add2/2(In2)
  From91/1 -> reset_out4/2, delayMatch8/1
  reset_out4/1 -> psi_1/1, delayMatch7/1
  Divide2_outbuff/1 -> Add1/2(In2)
  From51/1 -> reset_out3/2, delayMatch6/1
  reset_out3/1 -> psi_/1, delayMatch5/1
  Divide_outbuff/1 -> Add/2(In2)
  From2/1 -> reset_out2/2, delayMatch4/1
  reset_out2/1 -> psi_d/1, delayMatch3/1
  Product_outbuff/1 -> Sum_stage3/2(In2)
  Product8_outbuff/1 -> Sum_stage2/2(In2)
  From31/1 -> reset_out/2, delayMatch2/1
  reset_out/1 -> psi_q/1, delayMatch1/1
  Product7_outbuff/1 -> Sum1_stage3/2(In2)
  Product1_outbuff/1 -> Sum1_stage2/2(In2)
  Gain_const9/1 -> Gain9/1(In1)
  Gain_const8/1 -> Gain8/1(In1)
  Gain_const7/1 -> Gain7/1(In1)
  Gain_const6/1 -> Gain6/1(In1)
  Gain_const5/1 -> Gain5/1(In1)
  Gain_const4/1 -> Gain4/1(In1)
  Gain_const3/1 -> Gain3/1(In1)
  Factor_const/1 -> Factor/1(In1)
  Gain_const2/1 -> Gain2/1(In1)
  Gain_const1/1 -> Gain1/1(In1)
  Gain_const/1 -> Gain/1(In1)
  t6/9 -> Demux1_mux_3/3
  t6/8 -> Demux1_mux_3/2
  t6/7 -> Demux1_mux_3/1
  t6/6 -> Demux1_mux_2/3
  t6/5 -> Demux1_mux_2/2
  t6/4 -> Demux1_mux_2/1
  t6/3 -> Demux1_mux_1/3
  t6/2 -> Demux1_mux_1/2
  t6/1 -> Demux1_mux_1/1
  Sum_stage2_outbuff/1 -> Sum_stage3/1(In1)
  Sum1_stage2_outbuff/1 -> Sum1_stage3/1(In1)
  t5/2 -> Goto12/1
  t5/1 -> Goto11/1
  t4/9 -> Add6/1(In1)
  t4/8 -> Add5/1(In1)
  t4/7 -> Add4/1(In1)
  t4/6 -> Add3/1(In1)
  t4/5 -> Add2/1(In1)
  t4/4 -> Add1/1(In1)
  t4/3 -> Add/1(In1)
  t4/2 -> Transformation_out1_1_wire/1
  t4/1 -> Transformation_out1_0_wire/1
  t3/3 -> mux1/9
  t3/2 -> mux1/8
  t3/1 -> mux1/7
  t2/3 -> mux1/6
  t2/2 -> mux1/5
  t2/1 -> mux1/4
  t1/3 -> mux1/3
  t1/2 -> mux1/2
  t1/1 -> mux1/1
  reset_in2/1 -> crp_out_delay3/1
  reset_in/1 -> crp_out_delay1/1
  Data Type Conversion34/1 -> t6/1
  Transformation1/1(out) -> Data Type Conversion34/1, Data Type Conversion51/1(In1)
  delayMatch62/1 -> Transformation1/1(in)
  delayMatch61/1 -> mux2/9
  delayMatch60/1 -> mux2/8
  delayMatch59/1 -> mux2/7
  delayMatch58/1 -> mux2/6
  delayMatch57/1 -> mux2/5
  delayMatch56/1 -> mux2/4
  delayMatch55/1 -> mux2/3
  delayMatch54/1 -> mux2/2
  Goto6/1 -> From81/1
  From71/1 -> mux2/1
  Goto5/1 -> From71/1
  Divide13_outbuff/1 -> delayMatch61/1, Divide12/2(In2)
  Data Type Conversion20_outbuff/1 -> Divide13/1(In1)
  psi_6/1 -> Data Type Conversion20/1(In1)
  Sum3_outbuff10/1 -> reset_in9/3
  Gain_outbuff9/1 -> Sum310/1(In1)
  Data Type Conversion30_outbuff/1 -> Gain9/2(In2)
  Add6_outbuff/1 -> Data Type Conversion30/1(In1)
  delayMatch52/1 -> Divide13/2(In2)
  Goto151/1 -> From211/1
  delayMatch53/1 -> Divide12/1(In1)
  Initial_Val9/1 -> reset_in9/1, reset_out9/1
  Divide11_outbuff/1 -> delayMatch60/1, Divide10/2(In2)
  Data Type Conversion19_outbuff/1 -> Divide11/1(In1)
  psi_5/1 -> Data Type Conversion19/1(In1)
  Sum3_outbuff9/1 -> reset_in8/3
  Gain_outbuff8/1 -> Sum39/1(In1)
  Data Type Conversion29_outbuff/1 -> Gain8/2(In2)
  Add5_outbuff/1 -> Data Type Conversion29/1(In1)
  delayMatch50/1 -> Divide11/2(In2)
  Goto141/1 -> From20/1
  delayMatch51/1 -> Divide10/1(In1)
  Initial_Val8/1 -> reset_in8/1, reset_out8/1
  Divide9_outbuff/1 -> delayMatch59/1, Divide8/2(In2)
  Data Type Conversion18_outbuff/1 -> Divide9/1(In1)
  psi_4/1 -> Data Type Conversion18/1(In1)
  Sum3_outbuff8/1 -> reset_in7/3
  Gain_outbuff7/1 -> Sum38/1(In1)
  Data Type Conversion28_outbuff/1 -> Gain7/2(In2)
  Add4_outbuff/1 -> Data Type Conversion28/1(In1)
  delayMatch48/1 -> Divide9/2(In2)
  Goto131/1 -> From17/1
  delayMatch49/1 -> Divide8/1(In1)
  Initial_Val7/1 -> reset_in7/1, reset_out7/1
  Divide7_outbuff/1 -> delayMatch58/1, Divide6/2(In2)
  Data Type Conversion17_outbuff/1 -> Divide7/1(In1)
  psi_3/1 -> Data Type Conversion17/1(In1)
  Sum3_outbuff7/1 -> reset_in6/3
  Gain_outbuff6/1 -> Sum37/1(In1)
  Data Type Conversion27_outbuff/1 -> Gain6/2(In2)
  Add3_outbuff/1 -> Data Type Conversion27/1(In1)
  delayMatch46/1 -> Divide7/2(In2)
  Goto121/1 -> From16/1
  delayMatch47/1 -> Divide6/1(In1)
  Initial_Val6/1 -> reset_in6/1, reset_out6/1
  Divide5_outbuff/1 -> delayMatch57/1, Divide4/2(In2)
  Data Type Conversion16_outbuff/1 -> Divide5/1(In1)
  psi_2/1 -> Data Type Conversion16/1(In1)
  Sum3_outbuff6/1 -> reset_in5/3
  Gain_outbuff5/1 -> Sum36/1(In1)
  Data Type Conversion26_outbuff/1 -> Gain5/2(In2)
  Add2_outbuff/1 -> Data Type Conversion26/1(In1)
  delayMatch44/1 -> Divide5/2(In2)
  Goto111/1 -> From13/1
  delayMatch45/1 -> Divide4/1(In1)
  Initial_Val5/1 -> reset_in5/1, reset_out5/1
  Divide3_outbuff/1 -> delayMatch56/1, Divide2/2(In2)
  Data Type Conversion15_outbuff/1 -> Divide3/1(In1)
  psi_1/1 -> Data Type Conversion15/1(In1)
  Sum3_outbuff5/1 -> reset_in4/3
  Gain_outbuff4/1 -> Sum35/1(In1)
  Data Type Conversion25_outbuff/1 -> Gain4/2(In2)
  Add1_outbuff/1 -> Data Type Conversion25/1(In1)
  delayMatch42/1 -> Divide3/2(In2)
  Goto10/1 -> From121/1
  delayMatch43/1 -> Divide2/1(In1)
  Initial_Val4/1 -> reset_in4/1, reset_out4/1
  Divide1_outbuff/1 -> delayMatch55/1, Divide/2(In2)
  Data Type Conversion14_outbuff/1 -> Divide1/1(In1)
  psi_/1 -> Data Type Conversion141/1(In1)
  Sum3_outbuff4/1 -> reset_in3/3
  Gain_outbuff3/1 -> Sum34/1(In1)
  Data Type Conversion24_outbuff/1 -> Gain3/2(In2)
  Add_outbuff/1 -> Data Type Conversion24/1(In1)
  delayMatch40/1 -> Divide1/2(In2)
  Goto91/1 -> From111/1
  delayMatch41/1 -> Divide/1(In1)
  Goto32/1 -> From141/1, From181/1, From22/1, From26/1, From30/1, From41/1, From8/1
  Initial_Val3/1 -> reset_in3/1, reset_out3/1
  Goto2/1 -> From19/1
  Goto14/1 -> From18/1
  Goto7/1 -> From12/1
  Product9_outbuff/1 -> M_Mi/1
  Factor_outbuff/1 -> Product9/1(In1)
  Sum3_outbuff3/1 -> Factor/2(In2)
  Product2_outbuff/1 -> Sum33/2(In2)
  i_d/1 -> Goto5/1, Product2/1(In1)
  Data Type Conversion32_outbuff/1 -> i_d/1
  Product5_outbuff/1 -> Product8/1(In1), Data Type Conversion32/1(In1)
  Sum2_outbuff/1 -> Product5/2(In2)
  delayMatch29/1 -> Product1/2(In2)
  Sum3_outbuff2/1 -> reset_in2/3
  Gain_outbuff2/1 -> Sum32/1(In1)
  Sum_stage3_outbuff/1 -> Gain2/2(In2)
  Product10_outbuff/1 -> Product1/1(In1), Product/1(In1)
  Data Type Conversion33_outbuff1/1 -> Product10/1(In1)
  From61/1 -> Data Type Conversion331/1(In1)
  Goto4/1 -> From101/1, From61/1, From9/1
  Switch1/1 -> Goto4/1
  mechanical_system_out1/1 -> Switch1/1
  Data Type Conversion8_outbuff/1 -> mechanical_system_out1/1
  integrator_out1/1 -> Data Type Conversion81/1(In1)
  delayMatch31/1 -> Sum31/2(In2)
  Sum3_outbuff1/1 -> reset_in1/3
  Gain_outbuff1/1 -> Sum31/1(In1)
  Data Type Conversion1_outbuff/1 -> Gain1/2(In2)
  Product11_outbuff/1 -> Data Type Conversion14/1(In1)
  Sum1_outbuff/1 -> Product11/2(In2)
  delayMatch28/1 -> Product6/1(In1)
  Sum3_outbuff/1 -> reset_in/3
  Gain_outbuff/1 -> Sum3/1(In1)
  Sum1_stage3_outbuff/1 -> Gain/2(In2)
  Product6_outbuff/1 -> Data Type Conversion31/1(In1), Product7/1(In1)
  delayMatch37/1 -> Product2/2(In2)
  Data Type Conversion13_outbuff/1 -> pmsm_out4/1
  delayMatch38/1 -> Sum33/1(In1)
  delayMatch36/1 -> Product3/1(In1)
  Data Type Conversion23_outbuff/1 -> pmsm_out3/1
  i_q/1 -> Goto6/1, Product3/2(In2)
  Data Type Conversion31_outbuff/1 -> i_q/1
  delayMatch39/1 -> Product9/2(In2)
  Goto/1 -> From/1, From5/1
  From7/1 -> Product6/2(In2)
  Goto35/1 -> From7/1
  Initial_Val2/1 -> reset_in/1, reset_out/1
  Goto34/1 -> From6/1
  delayMatch27/1 -> Switch1/3
  Goto12/1 -> From21/1
  delayMatch26/1 -> Switch1/2
  Goto13/1 -> From14/1
  From1/1 -> Sum1/2(In2)
  Goto11/1 -> From1/1
  delayMatch30/1 -> Product11/1(In1)
  Goto3/1 -> From15/1
  bus_selector2/2 -> Goto3/1  "<1_J>"
  bus_selector2/1 -> Goto/1  "<polepair>"
  delayMatch32/1 -> reset_in1/2
  Initial_Val1/1 -> reset_in1/1, reset_out1/1
  Transformation_out1_1_wire/1 -> Goto2/1, Data Type Conversion22/1(In1)
  Transformation_out1_0_wire/1 -> Goto14/1, Data Type Conversion21/1(In1)
  Transformation/1(out) -> t4/1
  delayMatch23/1 -> Transformation/3(cos_theta_el)
  delayMatch22/1 -> Transformation/2(sin_theta_el)
  delayMatch25/1 -> Transformation/1(in)
  mux1/1 -> Data Type Conversion9/1(In1)
  Line-Line to Phase voltage2/1(Out1) -> t3/1
  Line-Line to Phase voltage1/1(Out1) -> t2/1
  Line-Line to Phase voltage/1(Out1) -> t1/1
  Goto1/1 -> From151/1, From191/1, From2/1, From23/1, From27/1, From31/1, From311/1, From51/1, From91/1
  From3/1 -> Goto1/1
  Goto9/1 -> From11/1, From131/1, From3/1, From4/1
  bus_selector1/2 -> Goto13/1  "<simulate_mechanical>"
  bus_selector1/1 -> Goto9/1  "<reset_integrators>"
  Initial_Val/1 -> reset_in2/1, reset_out2/1
  From24/1 -> Sum2/2(In2)
  Goto33/1 -> From24/1
  delayMatch34/1 -> Product5/1(In1)
  Goto36/1 -> From10/1
  bus_selector/12 -> Goto151/1  "<L_z3>"
  bus_selector/11 -> Goto141/1  "<L_y2>"
  bus_selector/10 -> Goto131/1  "<L_x2>"
  bus_selector/9 -> Goto121/1  "<L_y1>"
  bus_selector/8 -> Goto111/1  "<L_x1>"
  bus_selector/7 -> Goto10/1  "<L_z2>"
  bus_selector/6 -> Goto91/1  "<L_z1>"
  bus_selector/5 -> Data Type Conversion5/1(In1)  "<psi_pm>"
  bus_selector/4 -> Data Type Conversion3/1(In1)  "<polepair>"
  bus_selector/3 -> Goto32/1, Data Type Conversion33/1(In1)  "<R_1>"
  bus_selector/2 -> Data Type Conversion12/1(In1)  "<1_L_q>"
  bus_selector/1 -> Data Type Conversion11/1(In1)  "<1_L_d>"
  delayMatch21/1 -> Logical Operator/1
  From19/1 -> mux/5
  From18/1 -> mux/4
  delayMatch64/1 -> Wrapped State DTI/3(reset)
  delayMatch19/1 -> Wrapped State DTI/2(polepair)
  From101/1 -> Wrapped State DTI/1(Angular Speed)
  From9/1 -> mux/2
  From12/1 -> mux/1
  in17_repeat/1 -> reset_out9/3
  in16_repeat/1 -> reset_out8/3
  in15_repeat/1 -> reset_out7/3
  in14_repeat/1 -> reset_out6/3
  in13_repeat/1 -> reset_out5/3
  in12_repeat/1 -> reset_out4/3
  in11_repeat/1 -> reset_out3/3
  in10_repeat/1 -> reset_out2/3
  in9_repeat/1 -> reset_out1/3
  in8_repeat/1 -> Sum1/1(In1)
  in7_repeat/1 -> reset_out/3
  in6_repeat/1 -> t5/1
  in5_repeat/1 -> Data Type Conversion37/1(In1)
  in4_repeat/1 -> Cast To Double2/1(In1)
  in3_repeat/1 -> Cast To Double1/1(In1)
  in2_repeat/1 -> Cast To Double/1(In1)
  in1_repeat/1 -> bus_selector1/1
  in0_repeat/1 -> bus_selector/1, bus_selector2/1
  crp_out_delay14/1 -> Delay61/1
  crp_out_delay13/1 -> Delay51/1
  crp_out_delay12/1 -> Delay41/1
  crp_out_delay11/1 -> Delay1_lowered9/1
  crp_out_delay10/1 -> Delay1_lowered8/1
  crp_out_delay9/1 -> Delay1_lowered7/1
  crp_out_delay8/1 -> Delay1_lowered6/1
  crp_out_delay7/1 -> Delay1_lowered5/1
  crp_out_delay6/1 -> Delay1_lowered4/1
  crp_out_delay5/1 -> Delay1_lowered3/1
  crp_out_delay4/1 -> Delay8/1
  crp_out_delay3/1 -> Delay1_lowered2/1
  crp_out_delay2/1 -> Delay1_lowered1/1
  crp_out_delay1/1 -> Delay1_lowered/1
  Data Type Conversion1/1(Out1) -> crp_out_delay/1
  crp_out_delay/1 -> Delay7/1
  Data Type Conversion8/1 -> delayMatch/1
  mux/1 -> t/1
  Delay9/1 -> in3_repeat1/1
  Delay1_lowered9/1 -> in17_repeat/1
  Delay1_lowered8/1 -> in16_repeat/1
  Delay1_lowered7/1 -> in15_repeat/1
  Delay1_lowered6/1 -> in14_repeat/1
  Delay1_lowered5/1 -> in13_repeat/1
  Delay1_lowered4/1 -> in12_repeat/1
  Delay1_lowered3/1 -> in11_repeat/1
  Delay8/1 -> in8_repeat/1
  Delay1_lowered2/1 -> in10_repeat/1
  Delay1_lowered1/1 -> in9_repeat/1
  Delay1_lowered/1 -> in7_repeat/1
  delay/1 -> delayMatch70/1
  Delay6/1 -> delayMatch69/1
  Delay5/1 -> delayMatch68/1
  Delay4/1 -> delayMatch67/1
  t7/1 -> i_abc_ps/1
  t/1 -> outputs/1
  Wrapped State DTI/1(Angular Position) -> Data Type Conversion1/1(In1), mux/3
  Delay7/1 -> delay/1
  Delay61/1 -> Delay6/1
  Delay51/1 -> Delay5/1
  Delay41/1 -> Delay4/1
  delayMatch69/1 -> i_abc3_pl/1
  delayMatch68/1 -> i_abc2_pl/1
  delayMatch67/1 -> i_abc1_pl/1
  Delay3/1 -> in4_repeat/1
  Delay2/1 -> in3_repeat/1
  Delay1/1 -> in5_repeat/1
  Delay/1 -> in2_repeat/1
  delayMatch/1 -> in1_repeat1/1
  delayMatch70/1 -> out_theta_el/1
  pwm_trig/1 -> Data Type Conversion8/1
  in_theta_el/1 -> Delay1/1
  u_abc3_pl/1 -> Delay3/1
  u_abc2_pl/1 -> Delay2/1
  u_abc1_pl/1 -> Delay/1
  input/1 -> in6_repeat/1
  physical_parameters/1 -> in0_repeat/1
  Model_Parameter/1 -> in1_repeat/1

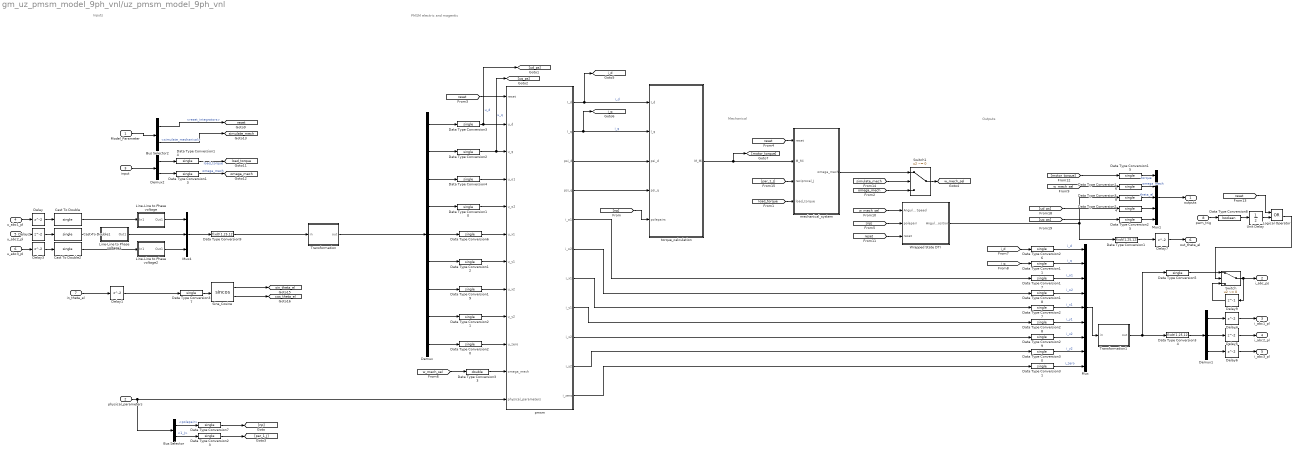
== system gm_uz_pmsm_model_9ph_vnl/uz_pmsm_model_9ph_vnl ==
  note: Inputs
  note: Outputs
  note: Mechanical
  note: PMSM electric and magentic
  Model_Parameter : Inport
  physical_parameters : Inport  Port=2
  input : Inport  Port=3
  u_abc1_pl : Inport  Port=4
  u_abc2_pl : Inport  Port=5
  u_abc3_pl : Inport  Port=6
  in_theta_el : Inport  Port=7
  pwm_trig : Inport  Port=8
  Bus Selector : BusSelector  OutputSignals=polepair,1_J
  Bus Selector2 : BusSelector  OutputSignals=reset_integrators,simulate_mechanical
  Cast To Double : DataTypeConversion  OutDataTypeStr=single
  Cast To Double1 : DataTypeConversion  OutDataTypeStr=single
  Cast To Double2 : DataTypeConversion  OutDataTypeStr=single
  Data Type Conversion1 : DataTypeConversion  OutDataTypeStr=fixdt(1,25,12)  RndMeth=Nearest
  Data Type Conversion{2..7,10..21,23..31,37..38} (29 alike) : DataTypeConversion  OutDataTypeStr=single  RndMeth=Nearest
  Data Type Conversion33 : DataTypeConversion  OutDataTypeStr=double  RndMeth=Nearest
  Data Type Conversion34 : DataTypeConversion  OutDataTypeStr=fixdt(1,25,12)  RndMeth=Nearest
  Data Type Conversion8 : DataTypeConversion  OutDataTypeStr=boolean  RndMeth=Nearest
  Data Type Conversion9 : DataTypeConversion  OutDataTypeStr=fixdt(1,25,12)  RndMeth=Nearest
  Delay{,1..7} (8 alike) : Delay
  Delay9 : Delay  DelayLength=1
  Demux : Demux  Outputs=9
  Demux1 : Demux  Outputs=3
  Demux2 : Demux  Outputs=2
  Line-Line to Phase voltage : Subsystem
  Line-Line to Phase voltage1 : Subsystem
  Line-Line to Phase voltage2 : Subsystem
  Logical Operator : Logic  Operator=OR  AllPortsSameDT=off  OutDataTypeStr=boolean
  Mux : Mux  Inputs=9
  Mux1 : Mux  Inputs=5
  Mux4 : Mux  Inputs=3
  Sine_Cosine : Trigonometry  Operator=sincos
  Switch : Switch  Criteria=u2 ~= 0
  Switch1 : Switch  Criteria=u2 ~= 0
  Transformation : Subsystem
  Transformation1 : Subsystem
  Unit Delay : UnitDelay  SampleTime=-1  HasFrameUpgradeWarning=on
  Wrapped State DTI : Subsystem
  mechanical_system : Subsystem
  pmsm : Subsystem
  torque_calculation : Subsystem
  outputs : Outport
  i_abc_ps : Outport  Port=2
  i_abc1_pl : Outport  Port=3
  i_abc2_pl : Outport  Port=4
  i_abc3_pl : Outport  Port=5
  out_theta_el : Outport  Port=6
  tag scope: cos_theta_el=global, i_d=global, i_q=global, load_torque=global, omega_mech=global, reset=global, simulate_mech=global, sin_theta_el=global, w_mech_sel=global
  wires:
  [reset] -> Logical Operator/1
  Logical Operator/1 -> Switch/2
  Unit Delay/1 -> Logical Operator/2
  Data Type Conversion8/1 -> Unit Delay/1
  pwm_trig/1 -> Data Type Conversion8/1
  Switch/1 -> Delay9/1, i_abc_ps/1
  Delay9/1 -> Switch/3
  Data Type Conversion5/1 -> Switch/1
  Sine_Cosine/2 -> [cos_theta_el]
  Sine_Cosine/1 -> [sin_theta_el]
  Delay3/1 -> Cast To Double2/1
  Delay2/1 -> Cast To Double1/1
  Line-Line to Phase voltage2/1(Out1) -> Mux4/3
  Cast To Double2/1 -> Line-Line to Phase voltage2/1(In1)
  Cast To Double1/1 -> Line-Line to Phase voltage1/1(In1)
  Line-Line to Phase voltage1/1(Out1) -> Mux4/2
  Line-Line to Phase voltage/1(Out1) -> Mux4/1
  Cast To Double/1 -> Line-Line to Phase voltage/1(In1)
  Delay/1 -> Cast To Double/1
  Delay1/1 -> Data Type Conversion37/1
  Data Type Conversion37/1 -> Sine_Cosine/1
  Data Type Conversion33/1 -> pmsm/11(omega_mech)
  [uq_ps] -> Data Type Conversion25/1
  [ud_ps] -> Data Type Conversion24/1
  Data Type Conversion25/1 -> Mux1/5
  Data Type Conversion24/1 -> Mux1/4
  Transformation/1(out) -> Demux/1
  Delay7/1 -> out_theta_el/1
  Delay6/1 -> i_abc3_pl/1
  Delay5/1 -> i_abc2_pl/1
  Delay4/1 -> i_abc1_pl/1
  Bus Selector/2 -> Data Type Conversion23/1  "<1_J>"
  Data Type Conversion23/1 -> [par_1_J]
  [w_mech_sel] -> Data Type Conversion33/1
  Data Type Conversion1/1 -> Delay7/1
  in_theta_el/1 -> Delay1/1
  [w_mech_sel] -> Wrapped State DTI/1(Angular Speed)
  Wrapped State DTI/1(Angular Position) -> Data Type Conversion1/1, Data Type Conversion38/1
  Demux1/2 -> Delay5/1
  Demux1/3 -> Delay6/1
  Demux1/1 -> Delay4/1
  Switch1/1 -> [w_mech_sel]
  Data Type Conversion34/1 -> Demux1/1
  Transformation1/1(out) -> Data Type Conversion5/1, Data Type Conversion34/1
  Mux/1 -> Transformation1/1(in)
  Mux1/1 -> outputs/1
  Data Type Conversion26/1 -> Mux/1  "i_d"
  Bus Selector2/2 -> [simulate_mech]  "<simulate_mechanical>"
  Bus Selector2/1 -> [reset]  "<reset_integrators>"
  Demux2/1 -> Data Type Conversion14/1
  Model_Parameter/1 -> Bus Selector2/1
  Mux4/1 -> Data Type Conversion9/1
  input/1 -> Demux2/1
  Data Type Conversion13/1 -> [omega_mech]  "omega_mech"
  Demux2/2 -> Data Type Conversion13/1
  u_abc3_pl/1 -> Delay3/1
  u_abc2_pl/1 -> Delay2/1
  Data Type Conversion9/1 -> Transformation/1(in)
  u_abc1_pl/1 -> Delay/1
  Data Type Conversion14/1 -> [load_torque]  "load_torque"
  [par_1_J] -> mechanical_system/3(reciprocal_J)
  Data Type Conversion7/1 -> [np]
  Bus Selector/1 -> Data Type Conversion7/1  "<polepair>"
  [motor_torque] -> Data Type Conversion15/1
  [reset] -> Wrapped State DTI/3(reset)
  [np] -> Wrapped State DTI/2(polepair)
  [w_mech_sel] -> Data Type Conversion16/1
  [i_d] -> Data Type Conversion26/1
  [i_q] -> Data Type Conversion11/1
  Data Type Conversion38/1 -> Mux1/3  "theta_el"
  pmsm/11(i_zero) -> Data Type Conversion31/1
  pmsm/10(i_y2) -> Data Type Conversion30/1
  pmsm/9(i_x2) -> Data Type Conversion29/1
  pmsm/8(i_y1) -> Data Type Conversion28/1
  pmsm/7(i_x1) -> Data Type Conversion27/1
  pmsm/6(i_o2) -> Data Type Conversion18/1
  Data Type Conversion21/1 -> pmsm/9(u_y2)
  [reset] -> mechanical_system/1(reset)
  [reset] -> pmsm/1(reset)
  Data Type Conversion31/1 -> Mux/9  "i_zero"
  Data Type Conversion30/1 -> Mux/8  "i_y2"
  Data Type Conversion29/1 -> Mux/7  "i_x2"
  Data Type Conversion28/1 -> Mux/6  "i_y1"
  Data Type Conversion27/1 -> Mux/5  "i_x1"
  pmsm/5(i_o1) -> Data Type Conversion17/1
  Data Type Conversion18/1 -> Mux/4  "i_o2"
  Data Type Conversion17/1 -> Mux/3  "i_o1"
  Data Type Conversion20/1 -> pmsm/10(u_zero)
  Data Type Conversion19/1 -> pmsm/8(u_x2)
  Data Type Conversion12/1 -> pmsm/7(u_y1)
  Data Type Conversion6/1 -> pmsm/6(u_x1)
  Data Type Conversion10/1 -> pmsm/5(u_o2)
  Data Type Conversion4/1 -> pmsm/4(u_o1)
  Demux/9 -> Data Type Conversion20/1
  Demux/8 -> Data Type Conversion21/1
  Demux/7 -> Data Type Conversion19/1
  Demux/6 -> Data Type Conversion12/1
  Demux/5 -> Data Type Conversion6/1
  Demux/4 -> Data Type Conversion10/1
  Demux/3 -> Data Type Conversion4/1
  [omega_mech] -> Switch1/3
  [load_torque] -> mechanical_system/4(load_torque)
  [np] -> torque_calculation/5(polepairs)
  Demux/2 -> Data Type Conversion2/1
  Demux/1 -> Data Type Conversion3/1
  Data Type Conversion11/1 -> Mux/2  "i_q"
  Data Type Conversion15/1 -> Mux1/1  "torque"
  Data Type Conversion16/1 -> Mux1/2  "omega_mech"
  pmsm/1(I_d) -> torque_calculation/1(I_d), [i_d]  "i_d"
  pmsm/2(I_q) -> torque_calculation/2(I_q), [i_q]  "i_q"
  mechanical_system/1(omega_mech) -> Switch1/1
  Data Type Conversion2/1 -> pmsm/3(u_q), [uq_ps]  "u_q"
  physical_parameters/1 -> Bus Selector/1, pmsm/12(physical_parameters)
  torque_calculation/1(M_Mi) -> mechanical_system/2(M_Mi), [motor_torque]
  [simulate_mech] -> Switch1/2
  Data Type Conversion3/1 -> pmsm/2(u_d), [ud_ps]  "u_d"
  pmsm/4(psi_q) -> torque_calculation/4(psi_q)
  pmsm/3(psi_d) -> torque_calculation/3(psi_d)
